simulink model "buck_boost_DCDC_realan_model_sim"  (R2020a)
settings: Solver=FixedStepAuto  StartTime=0.0  StopTime=sim_duration  FixedStep=time_step  RelTol=1e-3
undefined symbols (not defined in the file): beta, C, E, K_fl, K_smc_0, L, noise_enable, phi, prefiltar_enable, R, R_dot_enable, sigma_noise, step_poremecaj, step_ref, t_poremecaj, t_ref, time_step, w_diff, w_prefiltar, x_2e
libraries: powerlib x10, powerlib_meascontrol x1
settings Model: Creator=HP  LastModifiedBy=HP

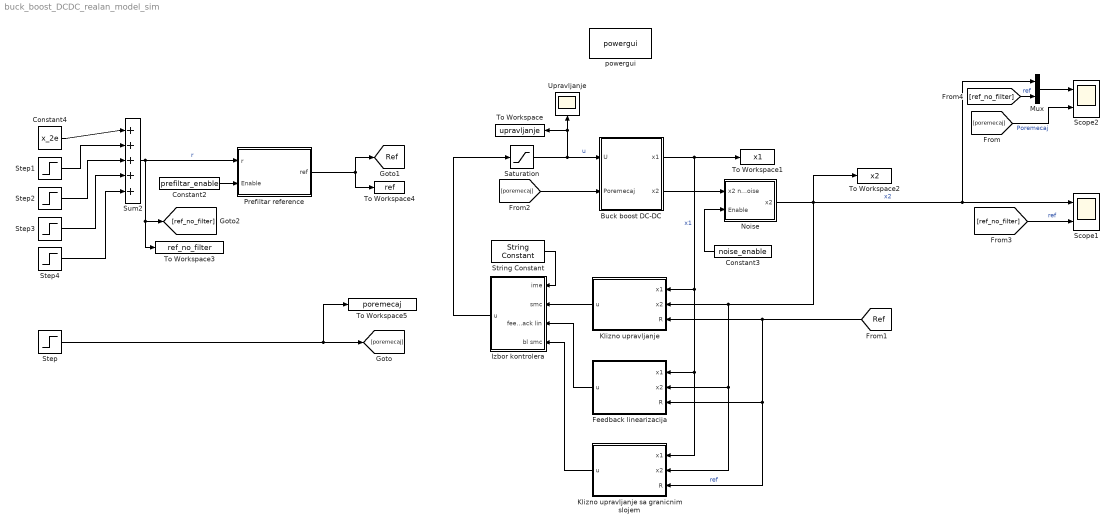
== system buck_boost_DCDC_realan_model_sim ==
  Buck boost DC-DC : Subsystem
  Constant2 : Constant  Value=prefiltar_enable
  Constant3 : Constant  Value=noise_enable
  Constant4 : Constant  Value=x_2e
  Feedback linearizacija : Subsystem
  Izbor kontrolera : Subsystem
  Klizno upravljanje : Subsystem
  Klizno upravljanje sa granicnim slojem : Subsystem
  Mux : Mux  Inputs=2
  Noise : Subsystem
  Prefiltar reference : Subsystem
  Saturation : Saturate  UpperLimit=1  LowerLimit=0
  Scope1 : Scope  NumInputPorts=2
  Scope2 : Scope  NumInputPorts=2
  Step : Step  Time=t_poremecaj(1)  After=step_poremecaj(1)  SampleTime=0
  Step1 : Step  Time=t_ref(1)  After=step_ref(1)  SampleTime=0
  Step2 : Step  Time=t_ref(2)  After=step_ref(2)  SampleTime=0
  Step3 : Step  Time=t_ref(3)  After=step_ref(3)  SampleTime=0
  Step4 : Step  Time=t_ref(4)  After=step_ref(4)  SampleTime=0
  String Constant : StringConstant  String=ime_kontrolera
  Sum2 : Sum  Inputs=|+++++
  To Workspace : ToWorkspace  VariableName=upravljanje  SaveFormat=Timeseries  SampleTime=-1
  To Workspace1 : ToWorkspace  VariableName=x1  SaveFormat=Timeseries  SampleTime=-1
  To Workspace2 : ToWorkspace  VariableName=x2  SaveFormat=Timeseries  SampleTime=-1
  To Workspace3 : ToWorkspace  VariableName=ref_no_filter  SaveFormat=Timeseries  SampleTime=-1
  To Workspace4 : ToWorkspace  VariableName=ref  SaveFormat=Timeseries  SampleTime=-1
  To Workspace5 : ToWorkspace  VariableName=poremecaj  SaveFormat=Timeseries  SampleTime=-1
  Upravljanje : Scope
  powergui : powerlib/powergui  Priority=1  SimulationMode=Continuous  SampleTime=50e-6  frequency=60  Iterations=50  frequencyindice=0  Pbase=100e6  ErrMax=1e-4  UnitsV=kV  UnitsW=MW  buscounter=0  FunctionMessages=off  echomessages=off  EnableUseOfTLC=off  CurrentSourceSwitches=off  DisableSnubberDevices=off  DisableRonSwitches=off  DisableVfSwitches=off  DisplayEquations=off  AutomaticDiscreteSolvers=off  SolverType=Tustin/Backward Euler (TBE)  Interpol=off  ExternalGateDelay=off  methode=off  Ts=100  x0status=blocks  SPID=on  SwTol=0  HookPort=off  NonlinearTolerance=1e-4  nMaxIteration=100  ContinueOnMaxIteration=off  RestoreLinks=warning  ResistiveCurrentMeasurement=off  Frange=[0:2:500]  Ylog=off  Xlog=on  ShowGrid=off  save=off  variable=ZData  structure=0  ZoomFFT=off  StartTime=0.0  cycles=1  DisplayStyle=1  fundamental=60  FreqAxis=off  MaxFrequency=1000  frequencyindicesteady=1  RmsSteady=1  display=off
  tag scope: Ref=global
  wires:
  Constant4/1 -> Sum2/1
  Saturation/1 -> To Workspace/1, Upravljanje/1, Buck boost DC-DC/1(U)  "u"
  Constant3/1 -> Noise/2(Enable)
  Constant2/1 -> Prefiltar reference/2(Enable)
  Prefiltar reference/1(ref) -> [Ref], To Workspace4/1
  Noise/1(x2) -> Mux/1, Scope1/1, To Workspace2/1, Klizno upravljanje sa granicnim slojem/2(x2), Feedback linearizacija/2(x2), Klizno upravljanje/2(x2)  "x2"
  Step/1 -> To Workspace5/1, [poremecaj]
  [ref_no_filter] -> Mux/2  "ref"
  Step3/1 -> Sum2/4
  Sum2/1 -> Prefiltar reference/1(r), [ref_no_filter], To Workspace3/1  "r"
  [poremecaj] -> Scope2/2  "Poremecaj"
  Feedback linearizacija/1(u) -> Izbor kontrolera/3(feedback lin)
  Step4/1 -> Sum2/5
  Klizno upravljanje sa granicnim slojem/1(u) -> Izbor kontrolera/4(bl smc)
  String Constant/1 -> Izbor kontrolera/1(ime)
  Klizno upravljanje/1(u) -> Izbor kontrolera/2(smc)
  Mux/1 -> Scope2/1
  Step1/1 -> Sum2/2
  [poremecaj] -> Buck boost DC-DC/2(Poremecaj)
  Step2/1 -> Sum2/3
  Buck boost DC-DC/2(x2) -> Noise/1(x2 no noise)
  [Ref] -> Klizno upravljanje sa granicnim slojem/3(R), Feedback linearizacija/3(R), Klizno upravljanje/3(R)  "ref"
  Buck boost DC-DC/1(x1) -> Klizno upravljanje sa granicnim slojem/1(x1), Feedback linearizacija/1(x1), Klizno upravljanje/1(x1), To Workspace1/1  "x1"
  Izbor kontrolera/1(u) -> Saturation/1
  [ref_no_filter] -> Scope1/2  "ref"

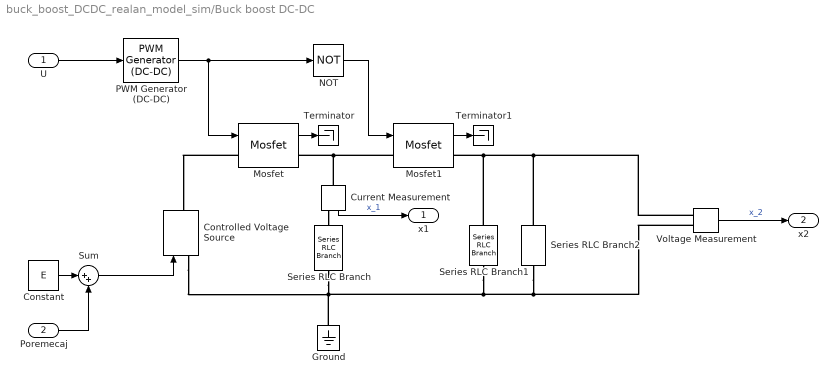
== system buck_boost_DCDC_realan_model_sim/Buck boost DC-DC ==
  U : Inport
  Poremecaj : Inport  Port=2
  Constant : Constant  Value=E
  Controlled Voltage Source : powerlib/Electrical Sources/Controlled Voltage Source  Initialize=on  Source_Type=AC  Amplitude=0  Phase=0  Frequency=0  Measurements=None
  Current Measurement : powerlib/Measurements/Current Measurement  PhasorSimulation=off  OutputType=Complex  PSBequivalent=0
  Ground : powerlib/Elements/Ground  LConnTagsString=a
  Mosfet : powerlib/Power Electronics/Mosfet  Ron=0.1  Lon=0  Rd=0.01  Vfd=0  IC=0  Rs=1e5  Cs=inf  Measurements=on
  Mosfet1 : powerlib/Power Electronics/Mosfet  Ron=0.1  Lon=0  Rd=0.01  Vfd=0  IC=0  Rs=1e5  Cs=inf  Measurements=on
  NOT : Logic  Operator=NOT  IconShape=distinctive  AllPortsSameDT=off  OutDataTypeStr=boolean
  PWM Generator (DC-DC) : powerlib_meascontrol/Pulse & Signal Generators/PWM Generator (DC-DC)  Fsw=f_sw  Ts=time_step
  Series RLC Branch : powerlib/Elements/Series RLC Branch  LConnTagsString=__new0  RConnTagsString=__new0  BranchType=L  Resistance=1  Inductance=L  SetiL0=off  InitialCurrent=0  Capacitance=1e-6  Setx0=off  InitialVoltage=0  Measurements=None
  Series RLC Branch1 : powerlib/Elements/Series RLC Branch  LConnTagsString=__new0  RConnTagsString=__new0  BranchType=C  Resistance=1  Inductance=1e-3  SetiL0=off  InitialCurrent=0  Capacitance=C  Setx0=off  InitialVoltage=0  Measurements=None
  Series RLC Branch2 : powerlib/Elements/Series RLC Branch  LConnTagsString=__new0  RConnTagsString=__new0  BranchType=R  Resistance=R  Inductance=L  SetiL0=off  InitialCurrent=0  Capacitance=1e-6  Setx0=off  InitialVoltage=0  Measurements=None
  Sum : Sum  Inputs=|++
  Terminator : Terminator
  Terminator1 : Terminator
  Voltage Measurement : powerlib/Measurements/Voltage Measurement  PhasorSimulation=off  OutputType=Complex  PSBequivalent=0
  x1 : Outport
  x2 : Outport  Port=2
  wires:
  Mosfet1/1 -> Terminator1/1
  PWM Generator (DC-DC)/1 -> Mosfet/1, NOT/1
  Mosfet/1 -> Terminator/1
  U/1 -> PWM Generator (DC-DC)/1
  NOT/1 -> Mosfet1/1
  Current Measurement/1 -> x1/1  "x_1"
  Voltage Measurement/1 -> x2/1  "x_2"
  Constant/1 -> Sum/1
  Sum/1 -> Controlled Voltage Source/1
  Poremecaj/1 -> Sum/2
  connections:
  Series RLC Branch/RConn1 -- Controlled Voltage Source/LConn1 -- Voltage Measurement/LConn2 -- Series RLC Branch2/RConn1 -- Series RLC Branch1/RConn1 -- Ground/LConn1
  Series RLC Branch1/LConn1 -- Voltage Measurement/LConn1 -- Series RLC Branch2/LConn1 -- Mosfet1/RConn1
  Mosfet1/LConn1 -- Current Measurement/LConn1 -- Mosfet/RConn1
  Mosfet/LConn1 -- Controlled Voltage Source/RConn1
  Current Measurement/RConn1 -- Series RLC Branch/LConn1

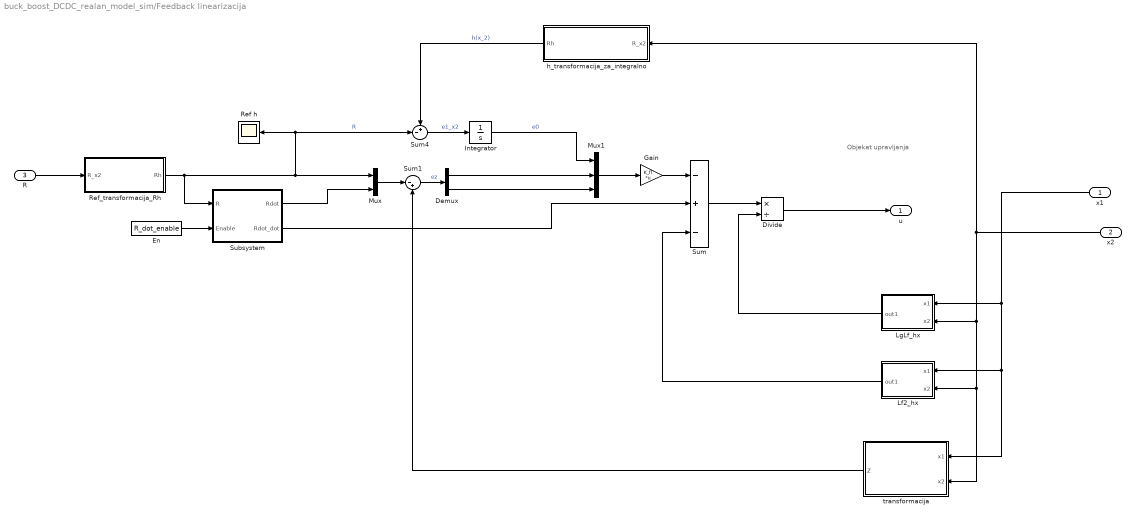
== system buck_boost_DCDC_realan_model_sim/Feedback linearizacija ==
  note: Objekat upravljanja
  x1 : Inport
  x2 : Inport  Port=2
  R : Inport  Port=3
  Demux : Demux  Outputs=2
  Divide : Product  Inputs=*/
  En : Constant  Value=R_dot_enable
  Gain : Gain  Gain=K_fl  Multiplication=Matrix(K*u)
  Integrator : Integrator
  Lf2_hx : MATLAB Function  TreatAsAtomicUnit=on
  LgLf_hx : MATLAB Function  TreatAsAtomicUnit=on
  Mux : Mux  Inputs=2
  Mux1 : Mux  Inputs=3
  Ref h : Scope
  Ref_transformacija_Rh : MATLAB Function  TreatAsAtomicUnit=on
  Subsystem : Subsystem
  Sum : Sum  Inputs=-+-
  Sum1 : Sum  Inputs=|-+
  Sum4 : Sum  Inputs=+-|
  h_transformacija_za_integralno : MATLAB Function  TreatAsAtomicUnit=on
  transformacija : MATLAB Function  TreatAsAtomicUnit=on
  u : Outport
  wires:
  Subsystem/1(Rdot) -> Mux/2
  Divide/1 -> u/1
  Ref_transformacija_Rh/1(Rh) -> Sum4/2, Ref h/1, Mux/1, Subsystem/1(R)  "R"
  x1/1 -> LgLf_hx/1(x1), Lf2_hx/1(x1), transformacija/1(x1)
  Mux/1 -> Sum1/1
  LgLf_hx/1(out1) -> Divide/2
  x2/1 -> h_transformacija_za_integralno/1(R_x2), LgLf_hx/2(x2), Lf2_hx/2(x2), transformacija/2(x2)
  Demux/1 -> Mux1/2
  Sum1/1 -> Demux/1  "ez"
  Gain/1 -> Sum/1
  Subsystem/2(Rdot_dot) -> Sum/2
  Lf2_hx/1(out1) -> Sum/3
  En/1 -> Subsystem/2(Enable)
  transformacija/1(Z) -> Sum1/2
  R/1 -> Ref_transformacija_Rh/1(R_x2)
  Sum/1 -> Divide/1
  Mux1/1 -> Gain/1
  Integrator/1 -> Mux1/1  "e0"
  Sum4/1 -> Integrator/1  "e1_x2"
  Demux/2 -> Mux1/3
  h_transformacija_za_integralno/1(Rh) -> Sum4/1  "h(x_2)"

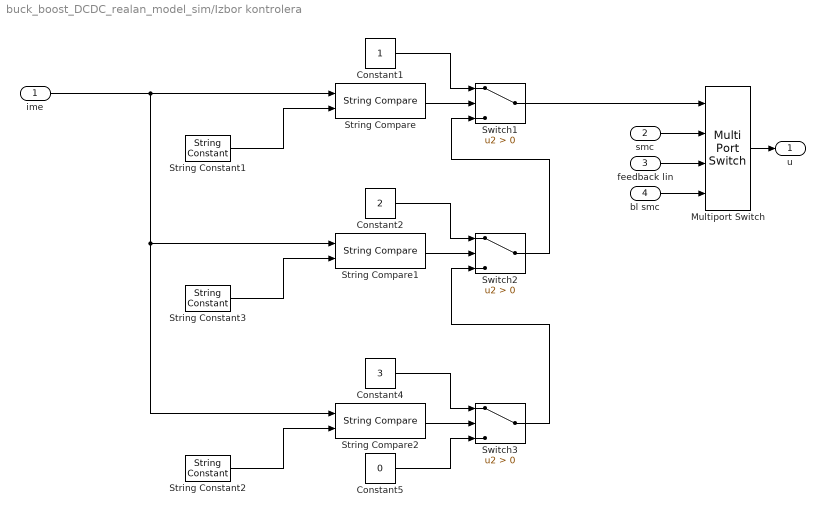
== system buck_boost_DCDC_realan_model_sim/Izbor kontrolera ==
  ime : Inport
  smc : Inport  Port=2
  feedback lin : Inport  Port=3
  bl smc : Inport  Port=4
  Constant1 : Constant
  Constant2 : Constant  Value=2
  Constant4 : Constant  Value=3
  Constant5 : Constant  Value=0
  Multiport Switch : MultiPortSwitch
  String Compare : StringCompare
  String Compare1 : StringCompare
  String Compare2 : StringCompare
  String Constant1 : StringConstant  String="\"smc\""
  String Constant2 : StringConstant  String="\"bl smc\""
  String Constant3 : StringConstant  String="\"fbl\""
  Switch1 : Switch  Criteria=u2 > Threshold
  Switch2 : Switch  Criteria=u2 > Threshold
  Switch3 : Switch  Criteria=u2 > Threshold
  u : Outport
  wires:
  String Compare1/1 -> Switch2/2
  Switch1/1 -> Multiport Switch/1
  String Constant1/1 -> String Compare/2
  String Constant3/1 -> String Compare1/2
  Constant1/1 -> Switch1/1
  Constant2/1 -> Switch2/1
  Switch2/1 -> Switch1/3
  String Compare/1 -> Switch1/2
  feedback lin/1 -> Multiport Switch/3
  Multiport Switch/1 -> u/1
  smc/1 -> Multiport Switch/2
  bl smc/1 -> Multiport Switch/4
  Constant5/1 -> Switch3/3
  ime/1 -> String Compare/1, String Compare2/1, String Compare1/1
  String Compare2/1 -> Switch3/2
  String Constant2/1 -> String Compare2/2
  Constant4/1 -> Switch3/1
  Switch3/1 -> Switch2/3

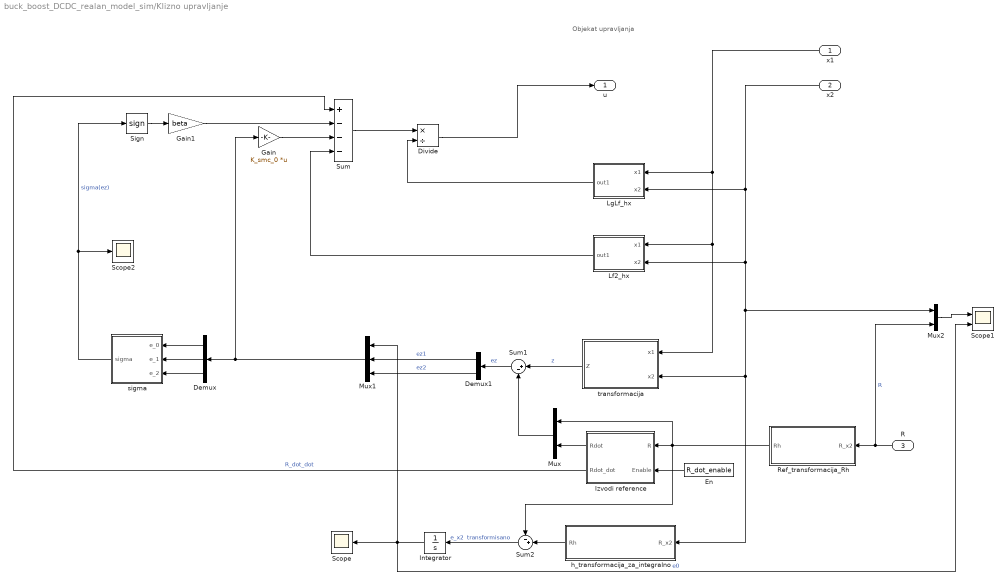
== system buck_boost_DCDC_realan_model_sim/Klizno upravljanje ==
  note: Objekat upravljanja
  x1 : Inport
  x2 : Inport  Port=2
  R : Inport  Port=3
  Demux : Demux  Outputs=3
  Demux1 : Demux  Outputs=2
  Divide : Product  Inputs=*/
  En : Constant  Value=R_dot_enable
  Gain : Gain  Gain=K_smc_0  Multiplication=Matrix(K*u)
  Gain1 : Gain  Gain=beta
  Integrator : Integrator
  Izvodi reference : Subsystem
  Lf2_hx : MATLAB Function  TreatAsAtomicUnit=on
  LgLf_hx : MATLAB Function  TreatAsAtomicUnit=on
  Mux : Mux  Inputs=2
  Mux1 : Mux  Inputs=3
  Mux2 : Mux  Inputs=2
  Ref_transformacija_Rh : MATLAB Function  TreatAsAtomicUnit=on
  Scope : Scope
  Scope1 : Scope  NumInputPorts=2
  Scope2 : Scope
  Sign : Signum
  Sum : Sum  Inputs=+---
  Sum1 : Sum  Inputs=|+-
  Sum2 : Sum  Inputs=-+|
  h_transformacija_za_integralno : MATLAB Function  TreatAsAtomicUnit=on
  sigma : MATLAB Function  TreatAsAtomicUnit=on
  transformacija : MATLAB Function  TreatAsAtomicUnit=on
  u : Outport
  wires:
  x1/1 -> LgLf_hx/1(x1), transformacija/1(x1), Lf2_hx/1(x1)
  x2/1 -> Mux2/1, h_transformacija_za_integralno/1(R_x2), transformacija/2(x2), Lf2_hx/2(x2), LgLf_hx/2(x2)
  Divide/1 -> u/1
  LgLf_hx/1(out1) -> Divide/2
  Sum/1 -> Divide/1
  Lf2_hx/1(out1) -> Sum/4
  Gain/1 -> Sum/3
  transformacija/1(Z) -> Sum1/1  "z"
  sigma/1(sigma) -> Sign/1, Scope2/1  "sigma(ez)"
  Sign/1 -> Gain1/1
  Gain1/1 -> Sum/2
  En/1 -> Izvodi reference/2(Enable)
  R/1 -> Mux2/2, Ref_transformacija_Rh/1(R_x2)  "R"
  Izvodi reference/1(Rdot) -> Mux/2
  Mux/1 -> Sum1/2
  Izvodi reference/2(Rdot_dot) -> Sum/1  "R_dot_dot"
  Ref_transformacija_Rh/1(Rh) -> Sum2/1, Mux/1, Izvodi reference/1(R)
  Mux1/1 -> Gain/1, Demux/1
  Sum1/1 -> Demux1/1  "ez"
  Demux1/1 -> Mux1/2  "ez1"
  Demux1/2 -> Mux1/3  "ez2"
  h_transformacija_za_integralno/1(Rh) -> Sum2/2
  Sum2/1 -> Integrator/1  "e_x2  transformisano"
  Demux/1 -> sigma/1(e_0)
  Demux/2 -> sigma/2(e_1)
  Demux/3 -> sigma/3(e_2)
  Integrator/1 -> Scope1/2, Scope/1, Mux1/1  "e0"
  Mux2/1 -> Scope1/1

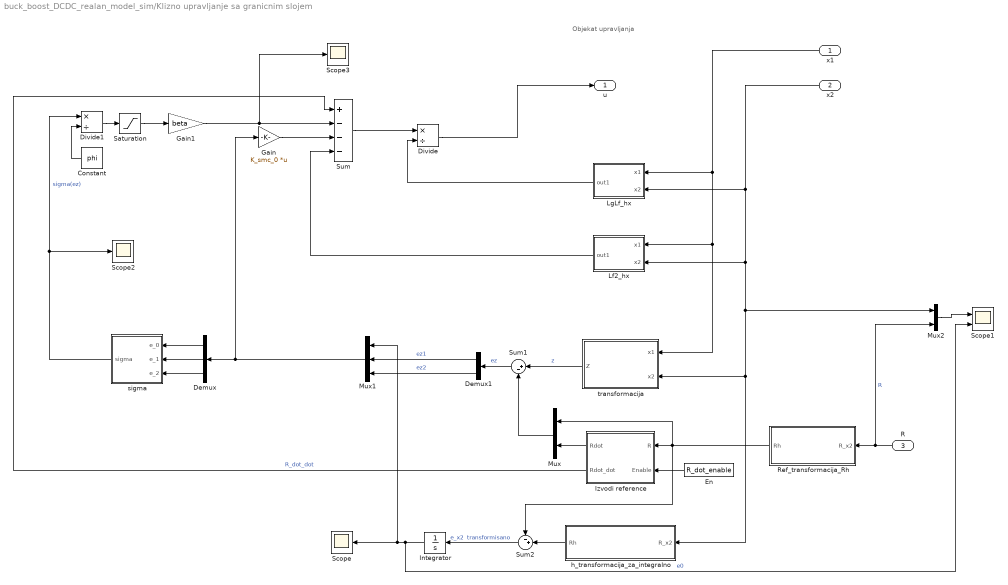
== system buck_boost_DCDC_realan_model_sim/Klizno upravljanje sa granicnim slojem ==
  note: Objekat upravljanja
  x1 : Inport
  x2 : Inport  Port=2
  R : Inport  Port=3
  Constant : Constant  Value=phi
  Demux : Demux  Outputs=3
  Demux1 : Demux  Outputs=2
  Divide : Product  Inputs=*/
  Divide1 : Product  Inputs=*/
  En : Constant  Value=R_dot_enable
  Gain : Gain  Gain=K_smc_0  Multiplication=Matrix(K*u)
  Gain1 : Gain  Gain=beta
  Integrator : Integrator
  Izvodi reference : Subsystem
  Lf2_hx : MATLAB Function  TreatAsAtomicUnit=on
  LgLf_hx : MATLAB Function  TreatAsAtomicUnit=on
  Mux : Mux  Inputs=2
  Mux1 : Mux  Inputs=3
  Mux2 : Mux  Inputs=2
  Ref_transformacija_Rh : MATLAB Function  TreatAsAtomicUnit=on
  Saturation : Saturate  UpperLimit=1  LowerLimit=-1
  Scope : Scope
  Scope1 : Scope  NumInputPorts=2
  Scope2 : Scope
  Scope3 : Scope
  Sum : Sum  Inputs=+---
  Sum1 : Sum  Inputs=|+-
  Sum2 : Sum  Inputs=-+|
  h_transformacija_za_integralno : MATLAB Function  TreatAsAtomicUnit=on
  sigma : MATLAB Function  TreatAsAtomicUnit=on
  transformacija : MATLAB Function  TreatAsAtomicUnit=on
  u : Outport
  wires:
  x1/1 -> LgLf_hx/1(x1), transformacija/1(x1), Lf2_hx/1(x1)
  x2/1 -> Mux2/1, h_transformacija_za_integralno/1(R_x2), transformacija/2(x2), Lf2_hx/2(x2), LgLf_hx/2(x2)
  Divide/1 -> u/1
  LgLf_hx/1(out1) -> Divide/2
  Sum/1 -> Divide/1
  Lf2_hx/1(out1) -> Sum/4
  Gain/1 -> Sum/3
  transformacija/1(Z) -> Sum1/1  "z"
  sigma/1(sigma) -> Divide1/1, Scope2/1  "sigma(ez)"
  Saturation/1 -> Gain1/1
  Gain1/1 -> Scope3/1, Sum/2
  En/1 -> Izvodi reference/2(Enable)
  R/1 -> Mux2/2, Ref_transformacija_Rh/1(R_x2)  "R"
  Izvodi reference/1(Rdot) -> Mux/2
  Mux/1 -> Sum1/2
  Izvodi reference/2(Rdot_dot) -> Sum/1  "R_dot_dot"
  Ref_transformacija_Rh/1(Rh) -> Sum2/1, Mux/1, Izvodi reference/1(R)
  Mux1/1 -> Gain/1, Demux/1
  Sum1/1 -> Demux1/1  "ez"
  Demux1/1 -> Mux1/2  "ez1"
  Demux1/2 -> Mux1/3  "ez2"
  h_transformacija_za_integralno/1(Rh) -> Sum2/2
  Sum2/1 -> Integrator/1  "e_x2  transformisano"
  Demux/1 -> sigma/1(e_0)
  Demux/2 -> sigma/2(e_1)
  Demux/3 -> sigma/3(e_2)
  Integrator/1 -> Scope1/2, Scope/1, Mux1/1  "e0"
  Mux2/1 -> Scope1/1
  Divide1/1 -> Saturation/1
  Constant/1 -> Divide1/2

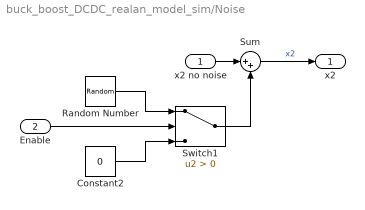
== system buck_boost_DCDC_realan_model_sim/Noise ==
  x2 no noise : Inport
  Enable : Inport  Port=2
  Constant2 : Constant  Value=0
  Random Number : RandomNumber  Variance=sigma_noise^2  SampleTime=time_step
  Sum : Sum  Inputs=|++
  Switch1 : Switch  Criteria=u2 > Threshold
  x2 : Outport
  wires:
  Random Number/1 -> Switch1/1
  Sum/1 -> x2/1  "x2"
  Switch1/1 -> Sum/2
  Enable/1 -> Switch1/2
  Constant2/1 -> Switch1/3
  x2 no noise/1 -> Sum/1

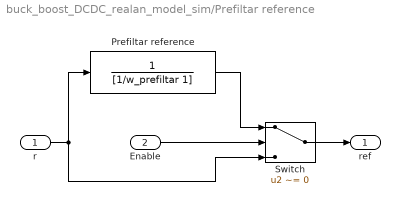
== system buck_boost_DCDC_realan_model_sim/Prefiltar reference ==
  r : Inport
  Enable : Inport  Port=2
  Prefiltar reference : TransferFcn  Denominator=[1/w_prefiltar 1]
  Switch : Switch  Criteria=u2 ~= 0
  ref : Outport
  wires:
  r/1 -> Switch/3, Prefiltar reference/1
  Enable/1 -> Switch/2
  Switch/1 -> ref/1
  Prefiltar reference/1 -> Switch/1

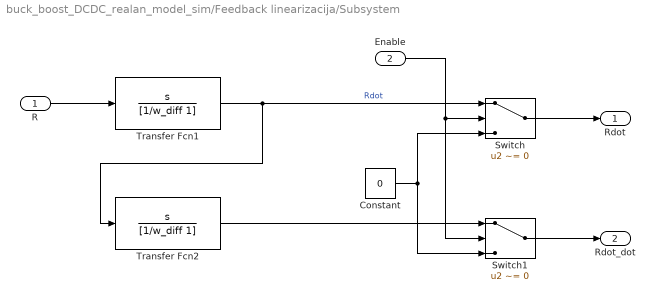
== system buck_boost_DCDC_realan_model_sim/Feedback linearizacija/Subsystem ==
  R : Inport
  Enable : Inport  Port=2
  Constant : Constant  Value=0
  Switch : Switch  Criteria=u2 ~= 0
  Switch1 : Switch  Criteria=u2 ~= 0
  Transfer Fcn1 : TransferFcn  Numerator=[1 0]  Denominator=[1/w_diff 1]
  Transfer Fcn2 : TransferFcn  Numerator=[1 0]  Denominator=[1/w_diff 1]
  Rdot : Outport
  Rdot_dot : Outport  Port=2
  wires:
  Transfer Fcn1/1 -> Switch/1, Transfer Fcn2/1  "Rdot"
  R/1 -> Transfer Fcn1/1
  Transfer Fcn2/1 -> Switch1/1
  Enable/1 -> Switch1/2, Switch/2
  Constant/1 -> Switch1/3, Switch/3
  Switch/1 -> Rdot/1
  Switch1/1 -> Rdot_dot/1

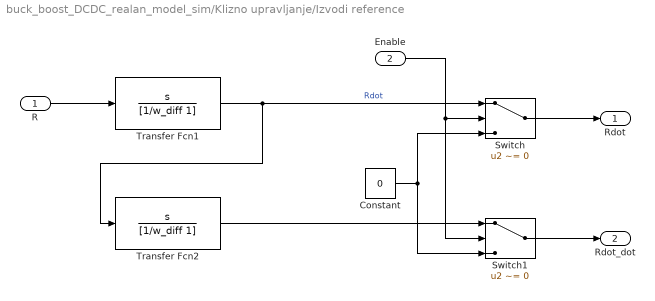
== system buck_boost_DCDC_realan_model_sim/Klizno upravljanje/Izvodi reference ==
  R : Inport
  Enable : Inport  Port=2
  Constant : Constant  Value=0
  Switch : Switch  Criteria=u2 ~= 0
  Switch1 : Switch  Criteria=u2 ~= 0
  Transfer Fcn1 : TransferFcn  Numerator=[1 0]  Denominator=[1/w_diff 1]
  Transfer Fcn2 : TransferFcn  Numerator=[1 0]  Denominator=[1/w_diff 1]
  Rdot : Outport
  Rdot_dot : Outport  Port=2
  wires:
  Transfer Fcn1/1 -> Switch/1, Transfer Fcn2/1  "Rdot"
  R/1 -> Transfer Fcn1/1
  Transfer Fcn2/1 -> Switch1/1
  Enable/1 -> Switch1/2, Switch/2
  Constant/1 -> Switch1/3, Switch/3
  Switch/1 -> Rdot/1
  Switch1/1 -> Rdot_dot/1

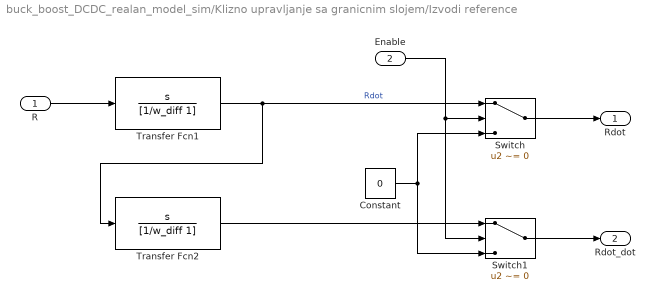
== system buck_boost_DCDC_realan_model_sim/Klizno upravljanje sa granicnim slojem/Izvodi reference ==
  R : Inport
  Enable : Inport  Port=2
  Constant : Constant  Value=0
  Switch : Switch  Criteria=u2 ~= 0
  Switch1 : Switch  Criteria=u2 ~= 0
  Transfer Fcn1 : TransferFcn  Numerator=[1 0]  Denominator=[1/w_diff 1]
  Transfer Fcn2 : TransferFcn  Numerator=[1 0]  Denominator=[1/w_diff 1]
  Rdot : Outport
  Rdot_dot : Outport  Port=2
  wires:
  Transfer Fcn1/1 -> Switch/1, Transfer Fcn2/1  "Rdot"
  R/1 -> Transfer Fcn1/1
  Transfer Fcn2/1 -> Switch1/1
  Enable/1 -> Switch1/2, Switch/2
  Constant/1 -> Switch1/3, Switch/3
  Switch/1 -> Rdot/1
  Switch1/1 -> Rdot_dot/1

== matlab function buck_boost_DCDC_realan_model_sim/Klizno upravljanje sa granicnim slojem/LgLf_hx ==
  data: x1 input; out1 output; x2 input
function out1 = LgLf_hx(x1,x2)
%#codegen

%    This function was generated by the Symbolic Math Toolbox version 8.5.
%    02-Jan-2021 23:18:57

out1 = x1.*9.819967266775777e+2-x2.*1.508485229415462e+3-x1.*x2.*1.636661211129296e+2+1.810182275298554e+4;

== matlab function buck_boost_DCDC_realan_model_sim/Klizno upravljanje sa granicnim slojem/Ref_transformacija_Rh ==
  data: R_x2 input; Rh output
function Rh = Ref_transformacija_Rh(R_x2)
%#codegen

%    This function was generated by the Symbolic Math Toolbox version 8.5.
%    02-Jan-2021 23:18:58

t2 = R_x2.^2;
Rh = R_x2.*(-1.128e-2)+t2.*4.7e-4+(R_x2.*1.2e+1-t2).^2.*4.086024819197896e-8-5.163584171453171e-1;

== matlab function buck_boost_DCDC_realan_model_sim/Klizno upravljanje sa granicnim slojem/h_transformacija_za_integralno ==
  data: R_x2 input; Rh output
function Rh = h_transformacija_za_integralno(R_x2)
%#codegen

%    This function was generated by the Symbolic Math Toolbox version 8.5.
%    02-Jan-2021 23:18:58

t2 = R_x2.^2;
Rh = R_x2.*(-1.128e-2)+t2.*4.7e-4+(R_x2.*1.2e+1-t2).^2.*4.086024819197896e-8-5.163584171453171e-1;

== matlab function buck_boost_DCDC_realan_model_sim/Klizno upravljanje sa granicnim slojem/sigma ==
  data: sigma output; e_0 input; e_1 input; e_2 input
function sigma = sigma(e_0,e_1,e_2)
%#codegen

%    This function was generated by the Symbolic Math Toolbox version 8.5.
%    02-Jan-2021 23:18:57

sigma = e_0.*6.25e+4+e_1.*5.0e+2+e_2;

== matlab function buck_boost_DCDC_realan_model_sim/Klizno upravljanje sa granicnim slojem/transformacija ==
  data: Z output; x1 input; x2 input
function Z = transformacija(x1,x2)
%#codegen

%    This function was generated by the Symbolic Math Toolbox version 8.5.
%    02-Jan-2021 23:18:57

Z = [x2.*(-1.128e-2)+x1.^2.*1.591e-2+x2.^2.*4.7e-4-5.163584171453171e-1;(x2.*9.4e-4-1.128e-2).*(x1.*5.2e+1+x2).*(-4.091653027823241e+1)+x1.*x2.*2.0];

== matlab function buck_boost_DCDC_realan_model_sim/Feedback linearizacija/LgLf_hx ==
  data: x1 input; out1 output; x2 input
function out1 = LgLf_hx(x1,x2)
%#codegen

%    This function was generated by the Symbolic Math Toolbox version 8.5.
%    02-Jan-2021 23:18:53

out1 = x1.*9.819967266775777e+2-x2.*1.508485229415462e+3-x1.*x2.*1.636661211129296e+2+1.810182275298554e+4;

== matlab function buck_boost_DCDC_realan_model_sim/Feedback linearizacija/transformacija ==
  data: x1 input; Z output; x2 input
function Z = transformacija(x1,x2)
%#codegen

%    This function was generated by the Symbolic Math Toolbox version 8.5.
%    02-Jan-2021 23:18:52

Z = [x2.*(-1.128e-2)+x1.^2.*1.591e-2+x2.^2.*4.7e-4-5.163584171453171e-1;(x2.*9.4e-4-1.128e-2).*(x1.*5.2e+1+x2).*(-4.091653027823241e+1)+x1.*x2.*2.0];

== matlab function buck_boost_DCDC_realan_model_sim/Feedback linearizacija/Lf2_hx ==
  data: x1 input; out1 output; x2 input
function out1 = Lf2_hx(x1,x2)
%#codegen

%    This function was generated by the Symbolic Math Toolbox version 8.5.
%    02-Jan-2021 23:18:53

out1 = x2.*1.508485229415462e+3+(x2./1.3e+1-6.0./1.3e+1).*(x1.*5.2e+1+x2).*4.091653027823241e+1;

== matlab function buck_boost_DCDC_realan_model_sim/Feedback linearizacija/Ref_transformacija_Rh ==
  data: R_x2 input; Rh output
function Rh = Ref_transformacija_Rh(R_x2)
%#codegen

%    This function was generated by the Symbolic Math Toolbox version 8.5.
%    02-Jan-2021 23:18:53

t2 = R_x2.^2;
Rh = R_x2.*(-1.128e-2)+t2.*4.7e-4+(R_x2.*1.2e+1-t2).^2.*4.086024819197896e-8-5.163584171453171e-1;

== matlab function buck_boost_DCDC_realan_model_sim/Feedback linearizacija/h_transformacija_za_integralno ==
  data: R_x2 input; Rh output
function Rh = h_transformacija_za_integralno(R_x2)
%#codegen

%    This function was generated by the Symbolic Math Toolbox version 8.5.
%    02-Jan-2021 23:18:53

t2 = R_x2.^2;
Rh = R_x2.*(-1.128e-2)+t2.*4.7e-4+(R_x2.*1.2e+1-t2).^2.*4.086024819197896e-8-5.163584171453171e-1;

== matlab function buck_boost_DCDC_realan_model_sim/Klizno upravljanje/transformacija ==
  data: Z output; x1 input; x2 input
function Z = transformacija(x1,x2)
%#codegen

%    This function was generated by the Symbolic Math Toolbox version 8.5.
%    02-Jan-2021 23:18:55

Z = [x2.*(-1.128e-2)+x1.^2.*1.591e-2+x2.^2.*4.7e-4-5.163584171453171e-1;(x2.*9.4e-4-1.128e-2).*(x1.*5.2e+1+x2).*(-4.091653027823241e+1)+x1.*x2.*2.0];

== matlab function buck_boost_DCDC_realan_model_sim/Klizno upravljanje/LgLf_hx ==
  data: x1 input; out1 output; x2 input
function out1 = LgLf_hx(x1,x2)
%#codegen

%    This function was generated by the Symbolic Math Toolbox version 8.5.
%    02-Jan-2021 23:18:55

out1 = x1.*9.819967266775777e+2-x2.*1.508485229415462e+3-x1.*x2.*1.636661211129296e+2+1.810182275298554e+4;

== matlab function buck_boost_DCDC_realan_model_sim/Klizno upravljanje/Lf2_hx ==
  data: x1 input; out1 output; x2 input
function out1 = Lf2_hx(x1,x2)
%#codegen

%    This function was generated by the Symbolic Math Toolbox version 8.5.
%    02-Jan-2021 23:18:55

out1 = x2.*1.508485229415462e+3+(x2./1.3e+1-6.0./1.3e+1).*(x1.*5.2e+1+x2).*4.091653027823241e+1;

== matlab function buck_boost_DCDC_realan_model_sim/Klizno upravljanje/sigma ==
  data: sigma output; e_0 input; e_1 input; e_2 input
function sigma = sigma(e_0,e_1,e_2)
%#codegen

%    This function was generated by the Symbolic Math Toolbox version 8.5.
%    02-Jan-2021 23:18:55

sigma = e_0.*6.25e+4+e_1.*5.0e+2+e_2;

== matlab function buck_boost_DCDC_realan_model_sim/Klizno upravljanje/Ref_transformacija_Rh ==
  data: R_x2 input; Rh output
function Rh = Ref_transformacija_Rh(R_x2)
%#codegen

%    This function was generated by the Symbolic Math Toolbox version 8.5.
%    02-Jan-2021 23:18:55

t2 = R_x2.^2;
Rh = R_x2.*(-1.128e-2)+t2.*4.7e-4+(R_x2.*1.2e+1-t2).^2.*4.086024819197896e-8-5.163584171453171e-1;

== matlab function buck_boost_DCDC_realan_model_sim/Klizno upravljanje/h_transformacija_za_integralno ==
  data: R_x2 input; Rh output
function Rh = h_transformacija_za_integralno(R_x2)
%#codegen

%    This function was generated by the Symbolic Math Toolbox version 8.5.
%    02-Jan-2021 23:18:55

t2 = R_x2.^2;
Rh = R_x2.*(-1.128e-2)+t2.*4.7e-4+(R_x2.*1.2e+1-t2).^2.*4.086024819197896e-8-5.163584171453171e-1;

== matlab function buck_boost_DCDC_realan_model_sim/Klizno upravljanje sa granicnim slojem/Lf2_hx ==
  data: x1 input; out1 output; x2 input
function out1 = Lf2_hx(x1,x2)
%#codegen

%    This function was generated by the Symbolic Math Toolbox version 8.5.
%    02-Jan-2021 23:18:57

out1 = x2.*1.508485229415462e+3+(x2./1.3e+1-6.0./1.3e+1).*(x1.*5.2e+1+x2).*4.091653027823241e+1;
